simulink model "simuEcuaDIf_Act4"  (R2019a)
settings: Solver=VariableStepAuto  StartTime=0.0  StopTime=10000  RelTol=1e-3
settings Model: Creator=pon_c  LastModifiedBy=pon_c

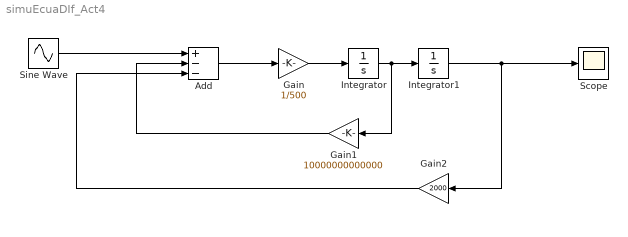
== system simuEcuaDIf_Act4 ==
  Add : Sum  Inputs=+--
  Gain : Gain  Gain=1/500
  Gain1 : Gain  Gain=10000000000000
  Gain2 : Gain  Gain=2000
  Integrator : Integrator
  Integrator1 : Integrator
  Scope : Scope
  Sine Wave : Sin  Amplitude=100  Frequency=3*pi  SampleTime=0
  wires:
  Gain/1 -> Integrator/1
  Add/1 -> Gain/1
  Integrator/1 -> Integrator1/1, Gain1/1
  Integrator1/1 -> Scope/1, Gain2/1
  Gain1/1 -> Add/2
  Gain2/1 -> Add/3
  Sine Wave/1 -> Add/1
